simulink model "TVModel_Simulation_21"  (R2021b)
settings: Solver=FixedStepDiscrete  StartTime=0.0  StopTime=250  FixedStep=0.02  MaxStep=0.01  RelTol=1e-3
undefined symbols (not defined in the file or in its folder): MB, TV, TV_OLD
libraries: simulink x22, simulink_extras x14, eeGeneralControl x13, slpidlib x8, fuzblock x4, controlLib x4, cstblocks x3, dspstat3 x2, eeSlidingModeController x1, sharedTrackingLibrary x1
(part 1 of 9)
settings Model: Creator=giuse  LastModifiedBy=Daniele
settings SolverCC: AutoInsertRateTranBlk=on
settings OptimizationCC: DefaultParameterBehavior=Inlined  UseDivisionForNetSlopeComputation=on  GainParamInheritBuiltInType=on  UseFloatMulNetSlope=on  InlineInvariantSignals=on  PassReuseOutputArgsAs=Individual arguments  ZeroExternalMemoryAtStartup=off  ZeroInternalMemoryAtStartup=off  NoFixptDivByZeroProtection=on  EfficientFloat2IntCast=on  LifeSpan=1  OptimizeBlockOrder=speed  DifferentSizesBufferReuse=on  EfficientTunableParamExpr=on
settings DebuggingCC: ParameterTunabilityLossMsg=error
settings HardwareCC: ProdBitPerPointer=32  ProdBitPerSizeT=32  ProdBitPerPtrDiffT=32  ProdLargestAtomicInteger=Long  ProdLargestAtomicFloat=Double  ProdWordSize=32  ProdLongLongMode=on  ProdHWDeviceType=ARM Compatible->ARM Cortex-M
settings SFSimCC: SimCustomHeaderCode="#include \"ITB_Nucleo_configuration\\Inc\\acados_wrapper.h\""  SimUserSources=ITB_Nucleo_configuration\Src\acados_wrapper.c  MATLABDynamicMemAlloc=off  CustomCodeUndefinedFunction=DoNotDetect
settings RTWCC: Description=Embedded Coder  SystemTargetFile=ert.tlc  GenCodeOnly=on  TemplateMakefile=ert_default_tmf  RTWUseSimCustomCode=on  CustomHeaderCode="#include \"ITB_Nucleo_configuration\\Inc\\acados_wrapper.h\""  CustomSource=ITB_Nucleo_configuration\Src\acados_wrapper.c
settings CodeAppCC: ForceParamTrailComments=on  IgnoreCustomStorageClasses=off  OperatorAnnotations=on  SimulinkDataObjDesc=on  SFDataObjDesc=on  CustomSymbolStrGlobalVar=rt$N$M  CustomSymbolStrType=$N$M  CustomSymbolStrFcn=$N$M$F  CustomSymbolStrMacro=$N$M  InsertBlockDesc=on
settings ERTTargetCC: TargetLangStandard=C99 (ISO)  GenerateSampleERTMain=on  IncludeMdlTerminateFcn=off  CombineSignalStateStructs=on  SupportAbsoluteTime=off  SupportComplex=off  SupportNonInlinedSFcns=on  InlinedParameterPlacement=NonHierarchical  ERTCustomFileTemplate=example_file_process.tlc  ERTFilePackagingFormat=CompactWithDataFile

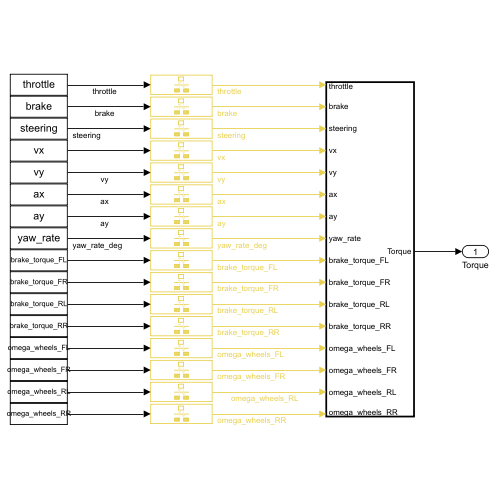
[thumbnail: Simulink's stored preview of the top-level diagram]
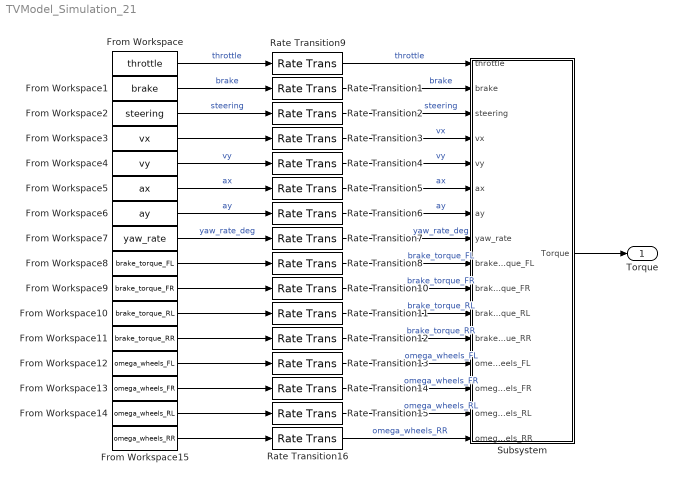
== system TVModel_Simulation_21 ==
  From Workspace : FromWorkspace  VariableName=throttle
  From Workspace1 : FromWorkspace  VariableName=brake
  From Workspace10 : FromWorkspace  VariableName=brake_torque_RL
  From Workspace11 : FromWorkspace  VariableName=brake_torque_RR
  From Workspace12 : FromWorkspace  VariableName=omega_wheels_FL
  From Workspace13 : FromWorkspace  VariableName=omega_wheels_FR
  From Workspace14 : FromWorkspace  VariableName=omega_wheels_RL
  From Workspace15 : FromWorkspace  VariableName=omega_wheels_RR
  From Workspace2 : FromWorkspace  VariableName=steering
  From Workspace3 : FromWorkspace  VariableName=vx
  From Workspace4 : FromWorkspace  VariableName=vy
  From Workspace5 : FromWorkspace  VariableName=ax
  From Workspace6 : FromWorkspace  VariableName=ay
  From Workspace7 : FromWorkspace  VariableName=yaw_rate
  From Workspace8 : FromWorkspace  VariableName=brake_torque_FL
  From Workspace9 : FromWorkspace  VariableName=brake_torque_FR
  Rate Transition{1..16} (16 alike) : RateTransition  OutPortSampleTime=TV.MPC.T/TV.MPC.N
  Subsystem : Subsystem  TreatAsAtomicUnit=on  PartitionName=Subsystem
  Torque : Outport
  wires:
  From Workspace4/1 -> Rate Transition4/1  "vy"
  From Workspace5/1 -> Rate Transition5/1  "ax"
  From Workspace1/1 -> Rate Transition1/1  "brake"
  From Workspace6/1 -> Rate Transition6/1  "ay"
  From Workspace10/1 -> Rate Transition11/1
  From Workspace11/1 -> Rate Transition12/1
  From Workspace15/1 -> Rate Transition16/1
  From Workspace12/1 -> Rate Transition13/1
  From Workspace9/1 -> Rate Transition10/1
  From Workspace7/1 -> Rate Transition7/1  "yaw_rate_deg"
  From Workspace13/1 -> Rate Transition14/1
  From Workspace14/1 -> Rate Transition15/1
  From Workspace2/1 -> Rate Transition2/1  "steering"
  From Workspace8/1 -> Rate Transition8/1
  From Workspace3/1 -> Rate Transition3/1
  From Workspace/1 -> Rate Transition9/1  "throttle"
  Subsystem/1(Torque) -> Torque/1
  Rate Transition9/1 -> Subsystem/1(throttle)  "throttle"
  Rate Transition1/1 -> Subsystem/2(brake)  "brake"
  Rate Transition2/1 -> Subsystem/3(steering)  "steering"
  Rate Transition3/1 -> Subsystem/4(vx)  "vx"
  Rate Transition4/1 -> Subsystem/5(vy)  "vy"
  Rate Transition5/1 -> Subsystem/6(ax)  "ax"
  Rate Transition6/1 -> Subsystem/7(ay)  "ay"
  Rate Transition7/1 -> Subsystem/8(yaw_rate)  "yaw_rate_deg"
  Rate Transition8/1 -> Subsystem/9(brake_torque_FL)  "brake_torque_FL"
  Rate Transition10/1 -> Subsystem/10(brake_torque_FR)  "brake_torque_FR"
  Rate Transition11/1 -> Subsystem/11(brake_torque_RL)  "brake_torque_RL"
  Rate Transition12/1 -> Subsystem/12(brake_torque_RR)  "brake_torque_RR"
  Rate Transition13/1 -> Subsystem/13(omega_wheels_FL)  "omega_wheels_FL"
  Rate Transition14/1 -> Subsystem/14(omega_wheels_FR)  "omega_wheels_FR"
  Rate Transition15/1 -> Subsystem/15(omega_wheels_RL)  "omega_wheels_RL"
  Rate Transition16/1 -> Subsystem/16(omega_wheels_RR)  "omega_wheels_RR"

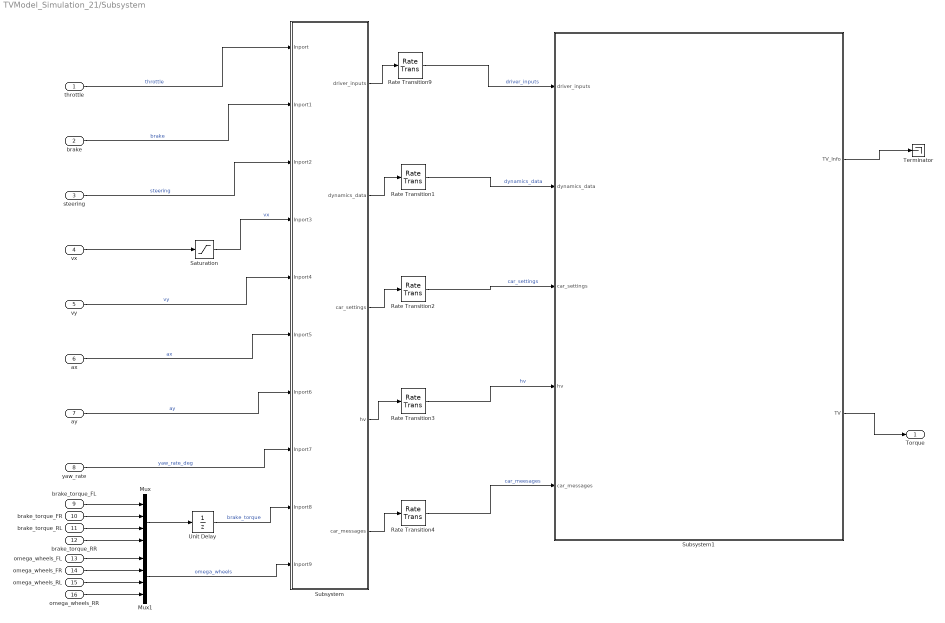
== system TVModel_Simulation_21/Subsystem ==
  throttle : Inport  SampleTime=0.02
  brake : Inport  Port=2
  steering : Inport  Port=3
  vx : Inport  Port=4
  vy : Inport  Port=5
  ax : Inport  Port=6
  ay : Inport  Port=7
  yaw_rate : Inport  Port=8
  brake_torque_FL : Inport  Port=9
  brake_torque_FR : Inport  Port=10
  brake_torque_RL : Inport  Port=11
  brake_torque_RR : Inport  Port=12
  omega_wheels_FL : Inport  Port=13
  omega_wheels_FR : Inport  Port=14
  omega_wheels_RL : Inport  Port=15
  omega_wheels_RR : Inport  Port=16
  Mux : Mux
  Mux1 : Mux
  Rate Transition{1..4,9} (5 alike) : RateTransition  OutPortSampleTime=TV.MPC.T/TV.MPC.N
  Saturation : Saturate  UpperLimit=inf  LowerLimit=0
  Subsystem : Subsystem
  Subsystem1 : Subsystem
  Terminator : Terminator
  Unit Delay : UnitDelay  SampleTime=-1  HasFrameUpgradeWarning=on
  Torque : Outport
  wires:
  omega_wheels_FL/1 -> Mux1/1
  ax/1 -> Subsystem/6(Inport5)  "ax"
  Unit Delay/1 -> Subsystem/9(Inport8)  "brake_torque"
  vy/1 -> Subsystem/5(Inport4)  "vy"
  ay/1 -> Subsystem/7(Inport6)  "ay"
  Mux1/1 -> Subsystem/10(Inport9)  "omega_wheels"
  Saturation/1 -> Subsystem/4(Inport3)  "vx"
  brake/1 -> Subsystem/2(Inport1)  "brake"
  yaw_rate/1 -> Subsystem/8(Inport7)  "yaw_rate_deg"
  throttle/1 -> Subsystem/1(Inport)  "throttle"
  brake_torque_RL/1 -> Mux/3
  vx/1 -> Saturation/1
  brake_torque_FL/1 -> Mux/1
  omega_wheels_RR/1 -> Mux1/4
  brake_torque_RR/1 -> Mux/4
  steering/1 -> Subsystem/3(Inport2)  "steering"
  omega_wheels_FR/1 -> Mux1/2
  Mux/1 -> Unit Delay/1
  omega_wheels_RL/1 -> Mux1/3
  brake_torque_FR/1 -> Mux/2
  Subsystem/1(driver_inputs) -> Rate Transition9/1
  Subsystem/2(dynamics_data) -> Rate Transition1/1
  Subsystem/5(car_messages) -> Rate Transition4/1
  Subsystem/3(car_settings) -> Rate Transition2/1
  Subsystem1/2(TV) -> Torque/1
  Subsystem1/1(TV_Info) -> Terminator/1
  Subsystem/4(hv) -> Rate Transition3/1
  Rate Transition9/1 -> Subsystem1/1(driver_inputs)  "driver_inputs"
  Rate Transition1/1 -> Subsystem1/2(dynamics_data)  "dynamics_data"
  Rate Transition2/1 -> Subsystem1/3(car_settings)  "car_settings"
  Rate Transition3/1 -> Subsystem1/4(hv)  "hv"
  Rate Transition4/1 -> Subsystem1/5(car_messages)  "car_meesages"

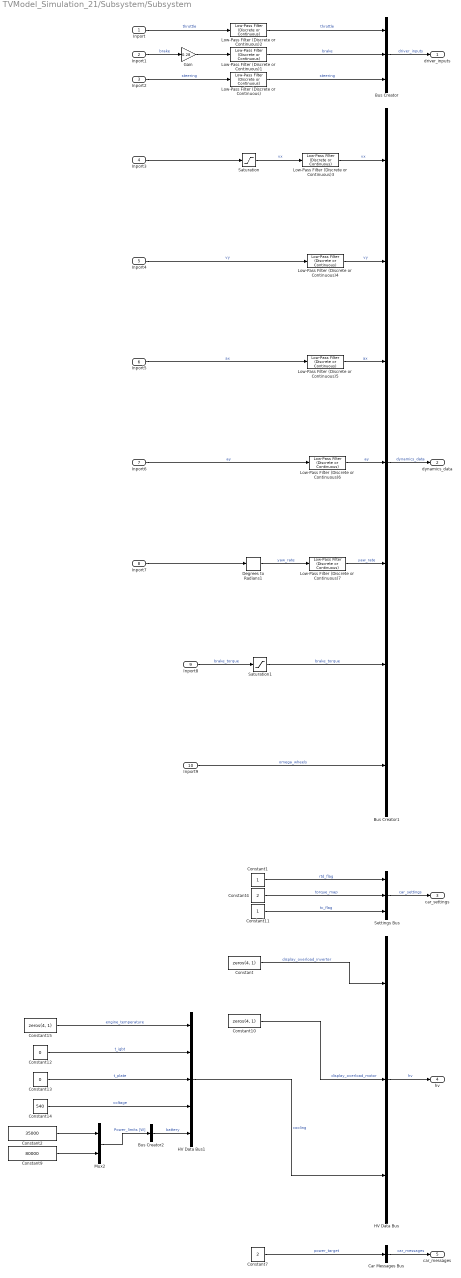
== system TVModel_Simulation_21/Subsystem/Subsystem ==
  Inport : Inport
  Inport1 : Inport  Port=2
  Inport2 : Inport  Port=3
  Inport3 : Inport  Port=4
  Inport4 : Inport  Port=5
  Inport5 : Inport  Port=6
  Inport6 : Inport  Port=7
  Inport7 : Inport  Port=8
  Inport8 : Inport  Port=9
  Inport9 : Inport  Port=10
  Bus Creator : BusCreator  Inputs=3
  Bus Creator1 : BusCreator  Inputs=7
  Bus Creator2 : BusCreator  Inputs=1
  Car Messages Bus : BusCreator  Inputs=1
  Constant : Constant  Value=zeros(4, 1)
  Constant1 : Constant  OutDataTypeStr=uint8
  Constant10 : Constant  Value=zeros(4, 1)
  Constant11 : Constant  OutDataTypeStr=uint8
  Constant12 : Constant  Value=0
  Constant13 : Constant  Value=0
  Constant14 : Constant  Value=540
  Constant15 : Constant  Value=zeros(4, 1)
  Constant2 : Constant  Value=35000
  Constant4 : Constant  Value=2  OutDataTypeStr=uint8
  Constant7 : Constant  Value=2
  Constant9 : Constant  Value=80000
  Degrees to Radians1 : simulink_extras/Transformations/Degrees to Radians
  Gain : Gain  Gain=0.28
  HV Data Bus : BusCreator  Inputs=3
  HV Data Bus1 : BusCreator  Inputs=5
  Low-Pass Filter (Discrete or Continuous) : eeGeneralControl/Low-Pass Filter (Discrete or Continuous)  K=1  T=1/(2*pi*1)  B=inf  A=-inf  init_option=Inherited from block input  x0=0  Ts=-1
  Low-Pass Filter (Discrete or Continuous)1 : eeGeneralControl/Low-Pass Filter (Discrete or Continuous)  K=1  T=1/(2*pi*10)  B=inf  A=-inf  init_option=Inherited from block input  x0=0  Ts=-1
  Low-Pass Filter (Discrete or Continuous)2 : eeGeneralControl/Low-Pass Filter (Discrete or Continuous)  K=1  T=1/(2*pi*10)  B=inf  A=-inf  init_option=Inherited from block input  x0=0  Ts=-1
  Low-Pass Filter (Discrete or Continuous){3..7} (5 alike) : eeGeneralControl/Low-Pass Filter (Discrete or Continuous)  K=1  T=1/(2*pi*3)  B=inf  A=-inf  init_option=Inherited from block input  x0=0  Ts=-1
  Mux2 : Mux  Inputs=2
  Saturation : Saturate  UpperLimit=inf  LowerLimit=0
  Saturation1 : Saturate  UpperLimit=inf  LowerLimit=0
  Settings Bus : BusCreator  Inputs=3
  driver_inputs : Outport
  dynamics_data : Outport  Port=2
  car_settings : Outport  Port=3
  hv : Outport  Port=4
  car_messages : Outport  Port=5
  wires:
  Constant4/1 -> Settings Bus/2  "torque_map"
  Inport2/1 -> Low-Pass Filter (Discrete or Continuous)/1  "steering"
  Constant1/1 -> Settings Bus/1  "rtd_flag"
  Car Messages Bus/1 -> car_messages/1  "car_messages"
  Inport9/1 -> Bus Creator1/7  "omega_wheels"
  Degrees to Radians1/1 -> Low-Pass Filter (Discrete or Continuous)7/1  "yaw_rate"
  Constant7/1 -> Car Messages Bus/1  "power_target"
  Bus Creator/1 -> driver_inputs/1  "driver_inputs"
  Inport7/1 -> Degrees to Radians1/1
  Settings Bus/1 -> car_settings/1  "car_settings"
  Bus Creator1/1 -> dynamics_data/1  "dynamics_data"
  Constant11/1 -> Settings Bus/3  "tc_flag"
  Inport6/1 -> Low-Pass Filter (Discrete or Continuous)6/1  "ay"
  Inport5/1 -> Low-Pass Filter (Discrete or Continuous)5/1  "ax"
  Inport4/1 -> Low-Pass Filter (Discrete or Continuous)4/1  "vy"
  Inport/1 -> Low-Pass Filter (Discrete or Continuous)2/1  "throttle"
  Inport8/1 -> Saturation1/1  "brake_torque"
  Inport1/1 -> Gain/1  "brake"
  Saturation/1 -> Low-Pass Filter (Discrete or Continuous)3/1  "vx"
  Inport3/1 -> Saturation/1
  HV Data Bus/1 -> hv/1  "hv"
  Mux2/1 -> Bus Creator2/1  "Power_limits [W]"
  Constant10/1 -> HV Data Bus/2  "display_overload_motor"
  HV Data Bus1/1 -> HV Data Bus/3  "cooling"
  Constant/1 -> HV Data Bus/1  "display_overload_inverter"
  Constant14/1 -> HV Data Bus1/4  "voltage"
  Constant12/1 -> HV Data Bus1/2  "t_igbt"
  Constant2/1 -> Mux2/1
  Constant13/1 -> HV Data Bus1/3  "t_plate"
  Constant9/1 -> Mux2/2
  Bus Creator2/1 -> HV Data Bus1/5  "battery"
  Constant15/1 -> HV Data Bus1/1  "engine_temperature"
  Low-Pass Filter (Discrete or Continuous)/1 -> Bus Creator/3  "steering"
  Low-Pass Filter (Discrete or Continuous)1/1 -> Bus Creator/2  "brake"
  Low-Pass Filter (Discrete or Continuous)2/1 -> Bus Creator/1  "throttle"
  Low-Pass Filter (Discrete or Continuous)3/1 -> Bus Creator1/1  "vx"
  Low-Pass Filter (Discrete or Continuous)4/1 -> Bus Creator1/2  "vy"
  Low-Pass Filter (Discrete or Continuous)5/1 -> Bus Creator1/3  "ax"
  Low-Pass Filter (Discrete or Continuous)6/1 -> Bus Creator1/4  "ay"
  Low-Pass Filter (Discrete or Continuous)7/1 -> Bus Creator1/5  "yaw_rate"
  Gain/1 -> Low-Pass Filter (Discrete or Continuous)1/1
  Saturation1/1 -> Bus Creator1/6  "brake_torque"

== system TVModel_Simulation_21/Subsystem/Subsystem1 ==
  In Bus Element2 : Inport  PortName=driver_inputs
  In Bus Element5 : Inport  PortName=driver_inputs
  In Bus Element11 : Inport  PortName=driver_inputs
  In Bus Element3 : Inport  Port=2  PortName=dynamics_data
  In Bus Element4 : Inport  Port=2  PortName=dynamics_data
  In Bus Element8 : Inport  Port=2  PortName=dynamics_data
  In Bus Element6 : Inport  Port=3  PortName=car_settings
  In Bus Element10 : Inport  Port=3  PortName=car_settings
  In Bus Element1 : Inport  Port=3  PortName=car_settings
  In Bus Element7 : Inport  Port=4  PortName=hv
  In Bus Element9 : Inport  Port=4  PortName=hv
  In Bus Element : Inport  Port=5  PortName=car_messages
  Slip Control : Subsystem
      settings: PortSchema="{\"entries\":[{\"content\":{\"sides\":[{\"content\":{\"connectorIds\":[\"In1\",\"In2\",\"In3\",\"In4\",\"In5\",\"In6\"]},\"type\":\"ConnectorPlacement.EquallySpacedRectSide\",\"uuid\":\"16d09c3a-8414-49ac-ac7a-3e724262c695\"},{\"content\":{\"connectorIds\":[\"Out1\",\"Out2\",\"Out3\"],\"side\":\"RIGHT\"},\"type\":\"ConnectorPlacement.EquallySpacedRectSide\",\"uuid\":\"762016d3-f980-4d0a-936f-11f940d81d21\"},{\"content\":{\"connectorIds\":[],\"side\":\"TOP\"},\"type\":\"ConnectorPlacement.EquallySpacedRectSide\",\"uuid\":\"9b181832-2af0-4676-9674-7a2572768951\"},{\"content\":{\"connectorIds\":[\"Out4\",\"Out5\"],\"side\":\"BOTTOM\"},\"type\":\"ConnectorPlacement.EquallySpacedRectSide\",\"uuid\":\"bd46a6db-b20b-4687-9f79-e5bb993d7a7e\"}]},\"type\":\"ConnectorPlacement.EquallySpacedConnector\",\"uuid\":\"fd23219d-68da-42e5-84a0-908c27a9841c\"}],\"packageUris\":[\"http://schema.mathworks.com/mf0/Connector/R2020b\"],\"version\":\"1.0\"}"
      mask Display: image('$imagefile'); % Use "Edit Image" on toolstrip to change.
  Terminator : Terminator
  Torque Distribution : Subsystem
      settings: PortSchema="{\"entries\":[{\"content\":{\"sides\":[{\"content\":{\"connectorIds\":[\"In1\",\"In2\",\"In3\",\"In4\",\"In5\",\"In6\",\"In7\",\"In8\",\"Out3\",\"In9\",\"In10\",\"In11\"]},\"type\":\"ConnectorPlacement.EquallySpacedRectSide\",\"uuid\":\"ece1a4aa-f225-4de9-8190-960458904133\"},{\"content\":{\"connectorIds\":[\"Out1\",\"Out2\"],\"side\":\"RIGHT\"},\"type\":\"ConnectorPlacement.EquallySpacedRectSide\",\"uuid\":\"588db727-2c2c-47b1-ab80-0176258858bf\"},{\"content\":{\"connectorIds\":[],\"side\":\"TOP\"},\"type\":\"ConnectorPlacement.EquallySpacedRectSide\",\"uuid\":\"54ce6245-2304-4750-b056-247655cbbdc1\"}]},\"type\":\"ConnectorPlacement.EquallySpacedConnector\",\"uuid\":\"9c8e646c-fa54-49ed-932c-87ddbb4d1884\"}],\"packageUris\":[\"http://schema.mathworks.com/mf0/Connector/R2020b\"],\"version\":\"1.0\"}"
      mask Display: image('$imagefile'); % Use "Edit Image" on toolstrip to change.
  Torque Limits : Subsystem
      mask Display: image('$imagefile'); % Use "Edit Image" on toolstrip to change.
  regen_brake : Subsystem
  steering_to_front_wheels : Subsystem
  Out Bus Element4 : Outport  PortName=TV_Info  Element=Torque_Distribution
  Out Bus Element6 : Outport  PortName=TV_Info  Element=Input_Signals.hv
  Out Bus Element7 : Outport  PortName=TV_Info  Element=Input_Signals.car_settings
  Out Bus Element8 : Outport  PortName=TV_Info  Element=Input_Signals.dynamics_data
  Out Bus Element9 : Outport  PortName=TV_Info  Element=Input_Signals.driver_inputs
  Out Bus Element10 : Outport  PortName=TV_Info  Element=Slip_Control
  Out Bus Element : Outport  Port=2  PortName=TV
  wires:
  In Bus Element4/1 -> Slip Control/2(dynamics_data)
  In Bus Element11/1 -> Slip Control/4(driver_inputs)
  In Bus Element5/1 -> Out Bus Element9/1  "driver_inputs"
  In Bus Element3/1 -> Torque Distribution/1(dynamics_data)
  Torque Distribution/3(TC_torque_out) -> Slip Control/6(tv)
  In Bus Element7/1 -> Out Bus Element6/1, Torque Limits/3(hv)
  Slip Control/1(TC_Torque) -> Torque Distribution/5(TC_Torque)
  steering_to_front_wheels/1(front_wheels_steering) -> Torque Distribution/4(front_wheels_steering), Slip Control/1(front_wheels_steering)
  Torque Limits/1(torque_limits) -> Slip Control/5(torque_limits), Torque Distribution/11(torque_limits)
  In Bus Element9/1 -> Torque Distribution/8(hv)
  Slip Control/4(slip_angles) -> Torque Distribution/10(slip_angles)
  In Bus Element6/1 -> Out Bus Element7/1, Torque Limits/2(car_settings)  "car_settings"
  Slip Control/2(slip_ratio) -> Torque Distribution/6(slip_ratio)
  Torque Distribution/2(TV) -> Out Bus Element/1
  In Bus Element1/1 -> Slip Control/3(car_settings)
  In Bus Element2/1 -> regen_brake/1(driver_inputs), Torque Distribution/2(driver_inputs), steering_to_front_wheels/1(driver_inputs)
  In Bus Element8/1 -> Torque Limits/1(dynamics_data), Out Bus Element8/1  "dynamics_data"
  regen_brake/1(brake_signal) -> Torque Distribution/3(brake_signal)
  In Bus Element/1 -> Terminator/1
  Slip Control/3(TV_Info) -> Out Bus Element10/1
  Torque Distribution/1(TV_info) -> Out Bus Element4/1
  Slip Control/5(Fz) -> Torque Distribution/9(Fz)
  In Bus Element10/1 -> Torque Distribution/7(Car_Settings)

== system TVModel_Simulation_21/Subsystem/Subsystem1/Slip Control ==
  In Bus Element6 : Inport  PortName=front_wheels_steering
  In Bus Element5 : Inport  PortName=front_wheels_steering
  In Bus Element10 : Inport  PortName=front_wheels_steering
  In Bus Element{1,3,8..9} (4 alike) : Inport  Port=2  PortName=dynamics_data
  In Bus Element2 : Inport  Port=3  PortName=car_settings
  In Bus Element4 : Inport  Port=4  PortName=driver_inputs
  In Bus Element : Inport  Port=5  PortName=torque_limits
  In Bus Element7 : Inport  Port=6  PortName=tv
  Load Transfer Calculation : Subsystem
  Slip Angle Calculation : Subsystem
  Slip Ratios : Subsystem
  Traction Control : Subsystem
  Out Bus Element1 : Outport  PortName=TC_Torque
  Out Bus Element : Outport  Port=2  PortName=slip_ratio
  Out Bus Element7 : Outport  Port=3  PortName=TV_Info  Element=Slip_Ratios
  Out Bus Element2 : Outport  Port=3  PortName=TV_Info  Element=Slip_Angles
  Out Bus Element3 : Outport  Port=3  PortName=TV_Info  Element=Fz
  Bus Element Out1 : Outport  Port=4  PortName=slip_angles
  Bus Element Out : Outport  Port=5  PortName=Fz
  wires:
  Slip Ratios/1(slip_ratio) -> Out Bus Element/1, Traction Control/3(slip_ratio)  "slip_ratio"
  In Bus Element1/1 -> Slip Ratios/1(dynamics_data)  "dynamics_data"
  In Bus Element6/1 -> Slip Ratios/2(front_wheels_steering)
  Slip Ratios/2(TV_Info) -> Out Bus Element7/1
  Traction Control/1(TC_Torque) -> Out Bus Element1/1
  In Bus Element2/1 -> Traction Control/2(car_settings)
  In Bus Element/1 -> Traction Control/4(torque_limits)
  In Bus Element7/1 -> Traction Control/1(tv)
  In Bus Element3/1 -> Traction Control/5(dynamics_data)
  In Bus Element4/1 -> Traction Control/7(driver_inputs)
  In Bus Element5/1 -> Traction Control/8(front_wheels_steering)
  In Bus Element8/1 -> Load Transfer Calculation/1(dynamics_data)
  In Bus Element10/1 -> Slip Angle Calculation/2(front_wheels_steering)
  Slip Angle Calculation/1(Slip angles [4x1]) -> Bus Element Out1/1, Traction Control/6(slip_angles)
  Slip Angle Calculation/2(TV_Info) -> Out Bus Element2/1
  In Bus Element9/1 -> Slip Angle Calculation/1(dynamics_data)
  Load Transfer Calculation/2(TV_Info) -> Out Bus Element3/1
  Load Transfer Calculation/1(Fz [4x1]) -> Traction Control/9(Fz), Bus Element Out/1

== system TVModel_Simulation_21/Subsystem/Subsystem1/Torque Distribution ==
  In Bus Element : Inport  PortName=dynamics_data
  In Bus Element1 : Inport  Port=2  PortName=driver_inputs
  In Bus Element9 : Inport  Port=2  PortName=driver_inputs
  In Bus Element3 : Inport  Port=3  PortName=brake_signal
  In Bus Element2 : Inport  Port=4  PortName=front_wheels_steering
  In Bus Element6 : Inport  Port=4  PortName=front_wheels_steering
  In Bus Element7 : Inport  Port=5  PortName=TC_Torque
  In Bus Element5 : Inport  Port=6  PortName=slip_ratio
  In Bus torque_map : Inport  Port=7  PortName=Car_Settings
  In Bus Element8 : Inport  Port=8  PortName=hv
  Bus Element In11 : Inport  Port=9  PortName=Fz
  Bus Element In : Inport  Port=10  PortName=slip_angles
  In Bus Element4 : Inport  Port=11  PortName=torque_limits
  MPC : Subsystem
      mask Display: image('$imagefile'); % Use "Edit Image" on toolstrip to change.
  Reference Tracking : Subsystem
      settings: PortSchema="{\"entries\":[{\"content\":{\"sides\":[{\"content\":{\"connectorIds\":[\"In1\",\"In2\",\"In3\"]},\"type\":\"ConnectorPlacement.EquallySpacedRectSide\",\"uuid\":\"f6b455b0-1993-4661-a7e5-67ec12298593\"},{\"content\":{\"connectorIds\":[\"Out1\"],\"side\":\"RIGHT\"},\"type\":\"ConnectorPlacement.EquallySpacedRectSide\",\"uuid\":\"cda4fcfc-381a-4065-8f38-4c677ea159cd\"},{\"content\":{\"connectorIds\":[\"Out2\"],\"side\":\"TOP\"},\"type\":\"ConnectorPlacement.EquallySpacedRectSide\",\"uuid\":\"ea61d581-e491-4d68-abf5-6728fc8d29b2\"}]},\"type\":\"ConnectorPlacement.EquallySpacedConnector\",\"uuid\":\"4f7fa02a-c913-4d0a-a26f-e6c9629c03da\"}],\"packageUris\":[\"http://schema.mathworks.com/mf0/Connector/R2020b\"],\"version\":\"1.0\"}"
      mask Display: image('$imagefile'); % Use "Edit Image" on toolstrip to change.
  Out Bus Element1 : Outport  PortName=TV_info  Element=MPC
  Out Bus Element : Outport  PortName=TV_info  Element=Reference
  Out Bus Element18 : Outport  Port=2  PortName=TV
  Out Bus Element2 : Outport  Port=3  PortName=TC_torque_out
  wires:
  In Bus torque_map/1 -> MPC/9(Car_Setting)
  In Bus Element5/1 -> MPC/4(slip_ratio)
  In Bus Element4/1 -> MPC/1(torque_limits)  "torque_limits_signals"
  In Bus Element3/1 -> MPC/7(brake_signal)  "regen"
  In Bus Element2/1 -> MPC/6(front_wheel_angles)  "front_wheels_steering_signals"
  Reference Tracking/1(yaw_rate_desired) -> MPC/3(yaw_rate_desired)  "yaw_rate_desired"
  In Bus Element/1 -> Reference Tracking/1(dynamics_data), MPC/2(dynamics_data)
  In Bus Element1/1 -> MPC/5(driver_inputs)  "driver_inputs_signals"
  In Bus Element6/1 -> Reference Tracking/2(front_wheels_steering)
  Reference Tracking/2(TV_Info) -> Out Bus Element/1
  MPC/1(TV_Info) -> Out Bus Element1/1
  In Bus Element7/1 -> MPC/8(TC_Torque)
  In Bus Element8/1 -> MPC/10(hv)  "hv"
  MPC/2(TV) -> Out Bus Element18/1
  MPC/3(TC_torque_out) -> Out Bus Element2/1
  In Bus Element9/1 -> Reference Tracking/3(driver_inputs)  "driver_inputs_signals"
  Bus Element In/1 -> MPC/11(slip_angles)
  Bus Element In11/1 -> MPC/12(Fz)

== system TVModel_Simulation_21/Subsystem/Subsystem1/Torque Limits ==
  In Bus Element6 : Inport  PortName=dynamics_data
  In Bus Element3 : Inport  PortName=dynamics_data
  In Bus torque_map1 : Inport  Port=2  PortName=car_settings
  In Bus torque_map2 : Inport  Port=2  PortName=car_settings
  In Bus Element2 : Inport  Port=3  PortName=hv
  In Bus Element1 : Inport  Port=3  PortName=hv
  Torque Limits Positive : Subsystem
  Torque Limits Regen : Subsystem
  Out Bus Element2 : Outport  PortName=torque_limits  Element=t_limit_positive
  Out Bus Element4 : Outport  PortName=torque_limits  Element=t_limit_negative
  wires:
  Torque Limits Regen/1(t_limit_regen) -> Out Bus Element4/1  "t_limit_negative"
  Torque Limits Positive/1(t_limit_positive) -> Out Bus Element2/1  "t_limit_positive"
  In Bus Element2/1 -> Torque Limits Positive/2(hv)  "hv"
  In Bus Element6/1 -> Torque Limits Positive/3(dynamics_data)  "omega_wheels"
  In Bus torque_map1/1 -> Torque Limits Positive/1(car_settings)  "torque_map"
  In Bus torque_map2/1 -> Torque Limits Regen/1(car_settings)  "torque_map"
  In Bus Element1/1 -> Torque Limits Regen/2(hv)  "hv"
  In Bus Element3/1 -> Torque Limits Regen/3(dynamics_data)  "omega_wheels"

== system TVModel_Simulation_21/Subsystem/Subsystem1/regen_brake ==
  In Bus Element : Inport  PortName=driver_inputs  Element=brake
  Gain : Gain  Gain=1/0.28
  Saturation : Saturate  UpperLimit=1  LowerLimit=0
  Out Bus Element : Outport  PortName=brake_signal  Element=regen
  wires:
  Gain/1 -> Saturation/1
  In Bus Element/1 -> Gain/1
  Saturation/1 -> Out Bus Element/1

== system TVModel_Simulation_21/Subsystem/Subsystem1/steering_to_front_wheels ==
  In Bus Element : Inport  PortName=driver_inputs  Element=steering
  In Bus Element1 : Inport  PortName=driver_inputs  Element=steering
  Abs : Abs
  Divide1 : Product  Inputs=**
  Mux : Mux  Inputs=2
  Sign : Signum
  Unary Minus : UnaryMinus
  steering_to_wheel_angle_single_axis_LUT : Lookup_n-D  NumberOfTableDimensions=1  BreakpointsForDimension1=TV.LUT.Car_LUT.steer_at_ground_single_axis_LUT.Steering  Table=TV.LUT.Car_LUT.steer_at_ground_single_axis_LUT.SteerAngle_SingleAxis  InternalRulePriority=Speed  RndMeth=Simplest  InputSameDT=on
  steering_to_wheel_angles_LUT : Lookup_n-D  NumberOfTableDimensions=1  BreakpointsForDimension1=TV.LUT.Car_LUT.steer_at_ground_LUT.Steering  Table=TV.LUT.Car_LUT.steer_at_ground_LUT.SteerAngle_FL  InternalRulePriority=Speed  RndMeth=Simplest  InputSameDT=on
  Out Bus Element : Outport  PortName=front_wheels_steering  Element=single_axis
  Out Bus Element1 : Outport  PortName=front_wheels_steering  Element=different_axis
  wires:
  Divide1/1 -> Out Bus Element1/1  "front_wheel_angle_single_axis_different_axis"
  steering_to_wheel_angle_single_axis_LUT/1 -> Out Bus Element/1  "front_wheel_angle_single_axis"
  Sign/1 -> Divide1/2
  Unary Minus/1 -> Mux/2
  In Bus Element/1 -> steering_to_wheel_angle_single_axis_LUT/1
  steering_to_wheel_angles_LUT/1 -> Abs/1  "front_wheel_angles"
  Mux/1 -> steering_to_wheel_angles_LUT/1
  Abs/1 -> Divide1/1
  In Bus Element1/1 -> Sign/1, Mux/1, Unary Minus/1

== system TVModel_Simulation_21/Subsystem/Subsystem1/Slip Control/Load Transfer Calculation ==
  In Bus Element : Inport  PortName=dynamics_data
  Fz FL : Subsystem
  Fz FR : Subsystem
  Fz RL : Subsystem
  Fz RR : Subsystem
  Mux : Mux
  Fz [4x1] : Outport
  Out Bus Element4 : Outport  Port=2  PortName=TV_Info  Element=fz_fl
  Out Bus Element1 : Outport  Port=2  PortName=TV_Info  Element=fz_fr
  Out Bus Element2 : Outport  Port=2  PortName=TV_Info  Element=fz_rl
  Out Bus Element3 : Outport  Port=2  PortName=TV_Info  Element=fz_rr
  wires:
  In Bus Element/1 -> Fz FL/1(dynamics_data), Fz FR/1(dynamics_data), Fz RL/1(dynamics_data), Fz RR/1(dynamics_data)
  Fz FL/1(TV_Info) -> Out Bus Element4/1, Mux/1  "Fz_FL"
  Fz FR/1(TV_Info) -> Mux/2, Out Bus Element1/1  "Fz_FR"
  Fz RL/1(TV_Info) -> Out Bus Element2/1, Mux/3  "Fz_RL"
  Fz RR/1(TV_Info) -> Out Bus Element3/1, Mux/4  "Fz_RR"
  Mux/1 -> Fz [4x1]/1

== system TVModel_Simulation_21/Subsystem/Subsystem1/Slip Control/Slip Angle Calculation ==
  In Bus Element{,2..4} (4 alike) : Inport  PortName=dynamics_data
  In Bus Element5 : Inport  PortName=dynamics_data  Element=vx
  In Bus Element10 : Inport  Port=2  PortName=front_wheels_steering
  In Bus Element1 : Inport  Port=2  PortName=front_wheels_steering
  Constant : Constant  Value=0
  Mux : Mux
  Slip Angle FL : Subsystem
  Slip Angle FR : Subsystem
  Slip Angle RL : Subsystem
  Slip Angle RR : Subsystem
  Switch : Switch  Criteria=u2 > Threshold  Threshold=3
  Slip angles [4x1] : Outport
  Out Bus Element4 : Outport  Port=2  PortName=TV_Info  Element=slip_angle_FL
  wires:
  Switch/1 -> Slip angles [4x1]/1, Out Bus Element4/1
  Slip Angle RR/1(alpha_rr) -> Mux/4  "alpha_rr"
  Slip Angle RL/1(alpha_rl) -> Mux/3  "alpha_rl"
  Slip Angle FR/1(alpha_fr) -> Mux/2  "alpha_fr"
  Slip Angle FL/1(alpha_fl) -> Mux/1  "alpha_fl"
  In Bus Element5/1 -> Switch/2
  Constant/1 -> Switch/3
  Mux/1 -> Switch/1
  In Bus Element4/1 -> Slip Angle RR/1(dynamics_data)
  In Bus Element3/1 -> Slip Angle RL/1(dynamics_data)
  In Bus Element2/1 -> Slip Angle FR/1(dynamics_data)
  In Bus Element1/1 -> Slip Angle FR/2(front_wheel_angles)
  In Bus Element10/1 -> Slip Angle FL/2(front_wheels_steering)
  In Bus Element/1 -> Slip Angle FL/1(dynamics_data)

== system TVModel_Simulation_21/Subsystem/Subsystem1/Slip Control/Slip Ratios ==
  In Bus Element{,2,4..5} (4 alike) : Inport  PortName=dynamics_data
  In Bus Element6 : Inport  Port=2  PortName=front_wheels_steering
  In Bus Element1 : Inport  Port=2  PortName=front_wheels_steering
  FL SR : Subsystem
  FR SR : Subsystem
  "RL RR " : Subsystem
  RL SR : Subsystem
  Out Bus Element : Outport  PortName=slip_ratio  Element=fl
  Out Bus Element1 : Outport  PortName=slip_ratio  Element=fr
  Out Bus Element2 : Outport  PortName=slip_ratio  Element=rl
  Out Bus Element3 : Outport  PortName=slip_ratio  Element=rr
  Out Bus Element4 : Outport  Port=2  PortName=TV_Info  Element=slip_ratio_fl
  Out Bus Element5 : Outport  Port=2  PortName=TV_Info  Element=slip_ratio_fr
  Out Bus Element6 : Outport  Port=2  PortName=TV_Info  Element=slip_ratio_rl
  Out Bus Element7 : Outport  Port=2  PortName=TV_Info  Element=slip_ratio_rr
  wires:
  In Bus Element5/1 -> "RL RR "/1(dynamics_data)
  In Bus Element4/1 -> RL SR/1(dynamics_data)
  In Bus Element2/1 -> FR SR/1(dynamics_data)
  In Bus Element1/1 -> FR SR/2(front_wheels_steering)
  In Bus Element6/1 -> FL SR/2(front_wheels_steering)
  In Bus Element/1 -> FL SR/1(dynamics_data)
  "RL RR "/1(RR) -> Out Bus Element7/1, Out Bus Element3/1  "kappa_RR"
  FR SR/1(FR) -> Out Bus Element5/1, Out Bus Element1/1  "kappa_FR"
  FL SR/1(FL) -> Out Bus Element4/1, Out Bus Element/1  "kappa_FL"
  RL SR/1(RL) -> Out Bus Element6/1, Out Bus Element2/1  "kappa_RL"

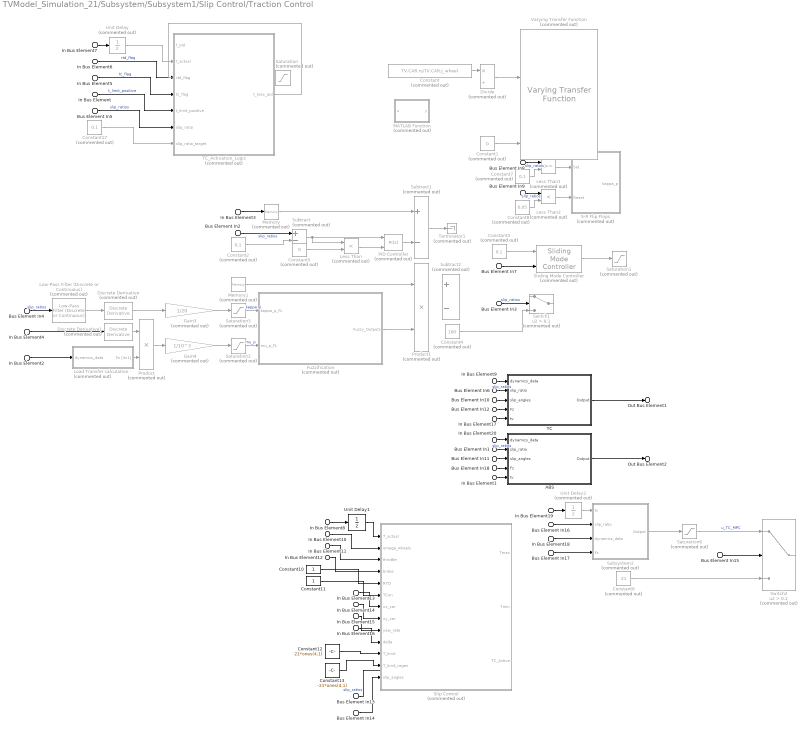
== system TVModel_Simulation_21/Subsystem/Subsystem1/Slip Control/Traction Control ==
  In Bus Element{1,3,7..8,17,19} (6 alike) : Inport  PortName=tv
  In Bus Element6 : Inport  Port=2  PortName=car_settings  Element=rtd_flag
  In Bus Element5 : Inport  Port=2  PortName=car_settings  Element=tc_flag
  Bus Element In{1..9,13,15..16} (12 alike) : Inport  Port=3  PortName=slip_ratio
  In Bus Element : Inport  Port=4  PortName=torque_limits  Element=t_limit_positive
  In Bus Element{2,9,18,20} (4 alike) : Inport  Port=5  PortName=dynamics_data
  In Bus Element4 : Inport  Port=5  PortName=dynamics_data  Element=ax
  In Bus Element10 : Inport  Port=5  PortName=dynamics_data  Element=omega_wheels
  In Bus Element13 : Inport  Port=5  PortName=dynamics_data  Element=vx
  In Bus Element14 : Inport  Port=5  PortName=dynamics_data  Element=vy
  In Bus Element15 : Inport  Port=5  PortName=dynamics_data  Element=yaw_rate
  Bus Element In10 : Inport  Port=6  PortName=slip_angles
  Bus Element In14 : Inport  Port=6  PortName=slip_angles
  Bus Element In11 : Inport  Port=6  PortName=slip_angles
  In Bus Element11 : Inport  Port=7  PortName=driver_inputs  Element=throttle
  In Bus Element12 : Inport  Port=7  PortName=driver_inputs  Element=brake
  In Bus Element16 : Inport  Port=8  PortName=front_wheels_steering  Element=single_axis
  Bus Element In12 : Inport  Port=9  PortName=Fz
  Bus Element In17 : Inport  Port=9  PortName=Fz
  Bus Element In18 : Inport  Port=9  PortName=Fz
  ABS : Subsystem
  Constant : Constant  Commented=on  Value=TV.CAR.rs/TV.CAR.J_wheel
  Constant1 : Constant  Commented=on  Value=0
  Constant10 : Constant
  Constant11 : Constant
  Constant12 : Constant  Value=21*ones(4,1)
  Constant13 : Constant  Value=-21*ones(4,1)
  Constant{2..3,7,17} (4 alike) : Constant  Commented=on  Value=0.1
  Constant4 : Constant  Commented=on  Value=100
  Constant5 : Constant  Commented=on  Value=0
  Constant6 : Constant  Commented=on  Value=21
  Constant8 : Constant  Commented=on  Value=0.05
  Discrete Derivative : simulink/Discrete/Discrete Derivative  Commented=on  gainval=1.0  ICPrevScaledInput=0.0  OutMin=[]  OutMax=[]  OutDataType=fixdt(1, 16)  OutScaling=2^-10  DoSatur=off
  Discrete Derivative1 : simulink/Discrete/Discrete Derivative  Commented=on  gainval=1.0  ICPrevScaledInput=0.0  OutMin=[]  OutMax=[]  OutDataType=fixdt(1, 16)  OutScaling=2^-10  DoSatur=off
  Divide : Product  Commented=on  Inputs=*/
  Fuzzification : Subsystem  Commented=on
  Gain3 : Gain  Commented=on  Gain=1/20
  Gain4 : Gain  Commented=on  Gain=1/10^3
  Less Than : RelationalOperator  Commented=on  Operator=<  OutDataTypeStr=boolean  RndMeth=Simplest
  Less Than1 : RelationalOperator  Commented=on  OutDataTypeStr=boolean  RndMeth=Simplest
  Less Than2 : RelationalOperator  Commented=on  Operator=<  OutDataTypeStr=boolean  RndMeth=Simplest
  Load Transfer calculation : Subsystem  Commented=on
  Low-Pass Filter (Discrete or Continuous) : eeGeneralControl/Low-Pass Filter (Discrete or Continuous)  Commented=on  K=1  T=1/(2*pi*3)  B=inf  A=-inf  init_option=Inherited from block input  x0=0  Ts=-1
  MATLAB Function : MATLAB Function  Commented=on  TreatAsAtomicUnit=on
  Memory : Memory  Commented=on  InheritSampleTime=on
  Memory1 : Memory  Commented=on  InheritSampleTime=on
  PID Controller : slpidlib/PID Controller  Commented=on  Controller=PI  Form=Parallel  TimeDomain=Discrete-time  UseExternalTs=off  SampleTime=-1  IntegratorMethod=Forward Euler  FilterMethod=Forward Euler  ControllerParametersSource=internal  P=2  I=5  D=0  UseFilter=on  N=100  TunerSelectOption=Transfer Function Based (PID Tuner App)  InitialConditionSource=internal  InitialConditionForIntegrator=0  InitialConditionForFilter=0  DifferentiatorICPrevScaledInput=0  ExternalReset=level  TrackingMode=off  Kt=1  LimitOutput=off  SatLimitsSource=internal  UpperSaturationLimit=inf  LowerSaturationLimit=-inf  LinearizeAsGain=on  AntiWindupMode=none  Kb=1  POutMin=[]  POutMax=[]  IOutMin=[]  IOutMax=[]  DOutMin=[]  DOutMax=[]  NOutMin=[]  NOutMax=[]  SumOutMin=[]  SumOutMax=[]  SaturationOutMin=[]  SaturationOutMax=[]  PParamMin=[]  PParamMax=[]  IParamMin=[]  IParamMax=[]  DParamMin=[]  DParamMax=[]  NParamMin=[]  NParamMax=[]  KbParamMin=[]  KbParamMax=[]  KtParamMin=[]  KtParamMax=[]  KbOutMin=[]  KbOutMax=[]  KtOutMin=[]  KtOutMax=[]  IntegratorOutMin=[]  IntegratorOutMax=[]  FilterOutMin=[]  FilterOutMax=[]  SumI1OutMin=[]  SumI1OutMax=[]  SumI2OutMin=[]  SumI2OutMax=[]  SumI3OutMin=[]  SumI3OutMax=[]  SumI4OutMin=[]  SumI4OutMax=[]  SumDOutMin=[]  SumDOutMax=[]  DifferentiatorOutMin=[]  DifferentiatorOutMax=[]  FilterDiffOutCoefMin=[]  FilterDiffOutCoefMax=[]  ReciprocalOutMin=[]  ReciprocalOutMax=[]  SumDenOutMin=[]  SumDenOutMax=[]  SumNumOutMin=[]  SumNumOutMax=[]  DivideOutMin=[]  DivideOutMax=[]  UdiffTsProdOutMin=[]  UdiffTsProdOutMax=[]  NTsProdOutMin=[]  NTsProdOutMax=[]  UintegralTsProdOutMin=[]  UintegralTsProdOutMax=[]  UngainTsProdOutMin=[]  UngainTsProdOutMax=[]  IntegratorContinuousStateAttributes=''  IntegratorStateMustResolveToSignalObject=off  IntegratorRTWStateStorageClass=Auto  FilterContinuousStateAttributes=''  FilterStateMustResolveToSignalObject=off  FilterRTWStateStorageClass=Auto  ParallelPVariant=InternalParameters  IdealPVariant=Disabled  IVariant=InternalParameters  DVariant=Disabled  IntegratorVariant=Discrete  SatVariant=Disabled  AWVariant=Passthrough  PCopyVariant=Disabled  TRVariant=Disabled  FdbkBlocksVariant=Forward  IdealPFdbkVariant=Disabled  SatFdbkVariant=Disabled  DerivativeFilterVariant=Disabled  NVariant=Disabled  NCopyVariant=Disabled_SignalSpec  FilterICVariant=Disabled  IntegratorICVariant=InternalICs  ExternalResetVariant=ExternalReset  TRSumVariant=Passthrough  SumFdbkVariant=Disabled  SumVariant=Sum_PI  TsampFilterVariant=InternalTs  TsampNgainVariant=Passthrough  TsampIntegralVariant=Passthrough  ExternalSaturationOutDataTypeStr=Inherit: Same as second input
  Product : Product  Commented=on
  Product1 : Product  Commented=on
  S-R Flip Flops : Subsystem  Commented=on
  Saturation : Saturate  Commented=on  UpperLimit=22  LowerLimit=0
  Saturation1 : Saturate  Commented=on  UpperLimit=inf  LowerLimit=0
  Saturation2 : Saturate  Commented=on  UpperLimit=1  LowerLimit=-1
  Saturation3 : Saturate  Commented=on  UpperLimit=1  LowerLimit=-1
  Saturation6 : Saturate  Commented=on  UpperLimit=21  LowerLimit=0
  Sliding Mode Controller : eeSlidingModeController/Sliding Mode Controller  Commented=on  h=0.2  up=10  lo=0  Ts=-1
      settings: SourceProductBaseCode=PS
  Slip Control : Subsystem  Commented=on
  Subsystem2 : Subsystem  Commented=on
  Subtract : Sum  Commented=on  Inputs=+-
  Subtract1 : Sum  Commented=on  Inputs=+-
  Subtract2 : Sum  Commented=on  Inputs=+-
  Switch1 : Switch  Commented=on  Criteria=u2 > Threshold  Threshold=0.1
  Switch2 : Switch  Commented=on  Criteria=u2 > Threshold  Threshold=0.1
  TC : Subsystem
  TC_Activation_Logic : Stateflow chart  Commented=on  TreatAsAtomicUnit=on
  Terminator1 : Terminator  Commented=on
  Unit Delay : UnitDelay  Commented=on  SampleTime=-1  HasFrameUpgradeWarning=on
  Unit Delay1 : UnitDelay  SampleTime=-1  HasFrameUpgradeWarning=on
  Unit Delay2 : UnitDelay  Commented=on  SampleTime=-1  HasFrameUpgradeWarning=on
  Varying Transfer Function : cstblocks/Linear Parameter Varying/Varying Transfer Function  Commented=on  N=1
  Out Bus Element1 : Outport  PortName=TC_Torque  Element=Traction
  Out Bus Element2 : Outport  PortName=TC_Torque  Element=Regen
  wires:
  In Bus Element1/1 -> ABS/5(tv)
  Bus Element In18/1 -> ABS/4(Fz)
  Bus Element In11/1 -> ABS/3(slip_angles)
  Bus Element In1/1 -> ABS/2(slip_ratio)  "slip_ratios"
  In Bus Element20/1 -> ABS/1(dynamics_data)
  Unit Delay2/1 -> Subsystem2/1(tv)
  In Bus Element18/1 -> Subsystem2/3(dynamics_data)
  Bus Element In17/1 -> Subsystem2/4(Fz)
  Bus Element In16/1 -> Subsystem2/2(slip_ratio)
  Subsystem2/1(Output) -> Saturation6/1
  In Bus Element19/1 -> Unit Delay2/1
  Subtract1/1 -> Terminator1/1
  Constant5/1 -> Less Than/2
  PID Controller/1 -> Subtract1/2
  Less Than/1 -> PID Controller/2
  Subtract/1 -> PID Controller/1, Less Than/1
  Low-Pass Filter (Discrete or Continuous)/1 -> Discrete Derivative/1
  Unit Delay/1 -> TC_Activation_Logic/2(t_actual)
  Constant17/1 -> TC_Activation_Logic/7(slip_ratio_target)
  Bus Element In5/1 -> TC_Activation_Logic/6(slip_ratio)  "slip_ratios"
  In Bus Element7/1 -> Unit Delay/1
  In Bus Element6/1 -> TC_Activation_Logic/3(rtd_flag)  "rtd_flag"
  In Bus Element5/1 -> TC_Activation_Logic/4(tc_flag)  "tc_flag"
  TC_Activation_Logic/1(t_max_pid) -> Saturation/1
  In Bus Element/1 -> TC_Activation_Logic/5(t_limit_positive)  "t_limit_positive"
  Constant/1 -> Divide/1
  Divide/1 -> Varying Transfer Function/2
  Constant1/1 -> Varying Transfer Function/4
  In Bus Element2/1 -> Load Transfer calculation/1(dynamics_data)
  Bus Element In2/1 -> Subtract/1  "slip_ratios"
  Bus Element In3/1 -> Switch1/2  "slip_ratios"
  In Bus Element3/1 -> Memory/1
  Memory/1 -> Subtract1/1
  Bus Element In7/1 -> Sliding Mode Controller/2
  Bus Element In4/1 -> Low-Pass Filter (Discrete or Continuous)/1  "slip_ratios"
  Constant3/1 -> Sliding Mode Controller/1
  Constant4/1 -> Switch1/3
  Discrete Derivative1/1 -> Product/1
  Discrete Derivative/1 -> Gain3/1
  Fuzzification/1(Fuzzy_Outputs) -> Product1/2
  Gain3/1 -> Saturation3/1
  Gain4/1 -> Saturation2/1
  In Bus Element4/1 -> Discrete Derivative1/1
  Load Transfer calculation/1(Fz [4x1]) -> Product/2
  Product/1 -> Gain4/1
  Saturation2/1 -> Fuzzification/2(mu_p_FL)  "mu_p"
  Saturation3/1 -> Fuzzification/1(kappa_p_FL)  "kappa_p"
  Sliding Mode Controller/1 -> Saturation1/1
  Constant2/1 -> Subtract/2
  Memory1/1 -> Product1/1
  In Bus Element9/1 -> TC/1(dynamics_data)
  Bus Element In6/1 -> TC/2(slip_ratio)  "slip_ratios"
  Bus Element In8/1 -> Less Than1/1  "slip_ratios"
  Constant7/1 -> Less Than1/2
  Less Than2/1 -> S-R Flip Flops/2(Reset)
  Bus Element In9/1 -> Less Than2/1  "slip_ratios"
  Less Than1/1 -> S-R Flip Flops/1(Set)
  Constant8/1 -> Less Than2/2
  In Bus Element10/1 -> Slip Control/2(omega_wheels)
  In Bus Element11/1 -> Slip Control/3(throttle)
  In Bus Element12/1 -> Slip Control/4(brake)
  Constant10/1 -> Slip Control/5(RTD)
  Constant11/1 -> Slip Control/6(TCon)
  In Bus Element13/1 -> Slip Control/7(vx_car)
  In Bus Element14/1 -> Slip Control/8(vy_car)
  In Bus Element15/1 -> Slip Control/9(yaw_rate)
  In Bus Element16/1 -> Slip Control/10(delta)
  Constant13/1 -> Slip Control/12(T_limit_regen)
  Constant12/1 -> Slip Control/11(T_limit)
  In Bus Element8/1 -> Unit Delay1/1
  Bus Element In10/1 -> TC/3(slip_angles)
  Bus Element In12/1 -> TC/4(Fz)
  Unit Delay1/1 -> Slip Control/1(T_actual)
  Bus Element In13/1 -> ?  "slip_ratios"
  Bus Element In14/1 -> Slip Control/13(slip_angles)
  In Bus Element17/1 -> TC/5(tv)
  Constant6/1 -> Switch2/3
  Saturation6/1 -> Switch2/1  "u_TC_MPC"
  Bus Element In15/1 -> Switch2/2
  TC/1(Output) -> Out Bus Element1/1
  ABS/1(Output) -> Out Bus Element2/1
